simulink model "rzs10thnew2021b"  (R2021b)
settings: Solver=FixedStepDiscrete  StartTime=0.0  StopTime=10.0  FixedStep=0.001  RelTol=1e-3  EnableMultiTasking=on
values from neighbouring files (symbols this model uses):
  F = 0.0    [rzdatabase.sldd]
  T = 1.0    [rzdatabase.sldd]
libraries: simulink x143, hdlsllib x95, spsEdgeDetectorLib x3
(part 1 of 3)
settings Model: DataDictionary=rzdatabase.sldd  Creator=icemi  LastModifiedBy=LENOVO
settings SolverCC: PositivePriorityOrder=on
settings OptimizationCC: DefaultParameterBehavior=Inlined  EnhancedBackFolding=on  PassReuseOutputArgsAs=Individual arguments  ZeroExternalMemoryAtStartup=off  ZeroInternalMemoryAtStartup=off  MaxStackSize=64  OptimizeBlockOrder=speed  DifferentSizesBufferReuse=on  OptimizationCustomize=off  EfficientTunableParamExpr=on
settings DebuggingCC: ParameterTunabilityLossMsg=error
settings HardwareCC: ProdBitPerPointer=32  ProdBitPerSizeT=32  ProdBitPerPtrDiffT=32  ProdLargestAtomicInteger=Long  ProdLargestAtomicFloat=Double  ProdWordSize=32  ProdHWDeviceType=NXP->Cortex-M4  HardwareBoardFeatureSet=SoCBlockset
settings ModelReferenceCC: ModelReferenceNumInstancesAllowed=Single
settings SFSimCC: MATLABDynamicMemAlloc=off
settings RTWCC: Description=Embedded Coder  SystemTargetFile=ert.tlc  PackageGeneratedCodeAndArtifacts=on  TemplateMakefile=ert_default_tmf
settings CodeAppCC: ForceParamTrailComments=on  IgnoreCustomStorageClasses=off  OperatorAnnotations=on  SimulinkDataObjDesc=on  SFDataObjDesc=on  InsertBlockDesc=on
settings ERTTargetCC: InlinedParameterPlacement=NonHierarchical  ERTCustomFileTemplate=example_file_process.tlc

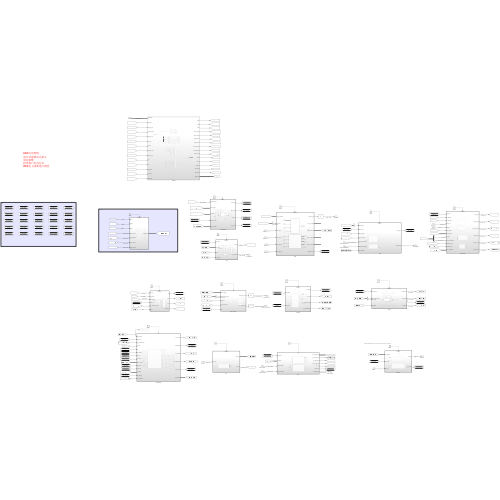
[thumbnail: Simulink's stored preview of the top-level diagram]
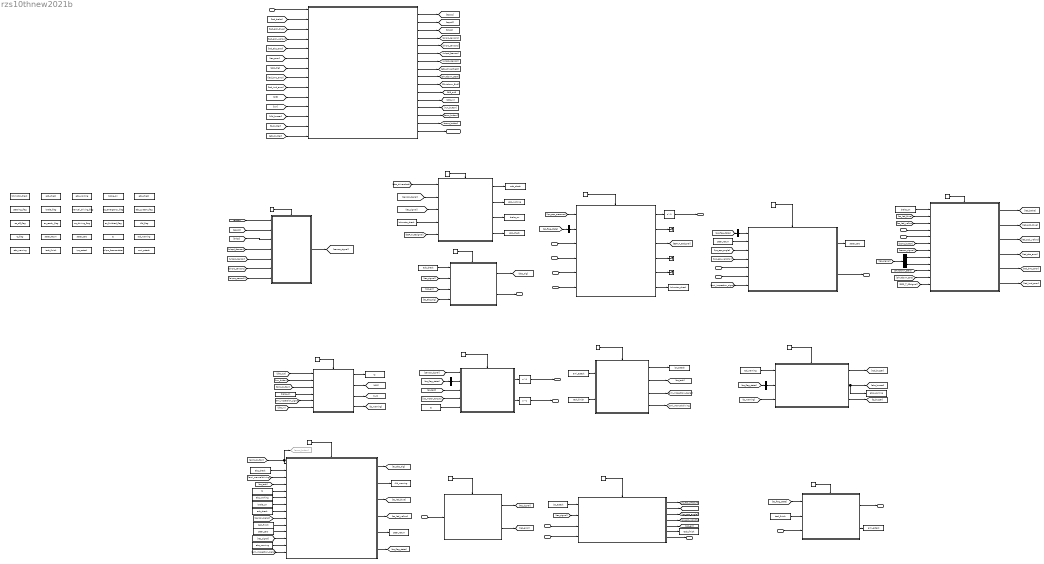
== system rzs10thnew2021b ==
  note: VCU发送状态机运行状态以及无人任务结束，接收无人任务选择
  note: EBS灯的逻辑
      | 油压传感器改为报文
      | 制动报警
      | 检查接口有没有多
      | RES定义重新建立模型
  note: 车身域
  note: 内存
  bms_error : Inport
  imd_error : Inport  Port=2
  ESP_T_01 : Inport  Port=3
  ESP_T_03 : Inport  Port=4
  ESP_T_06 : Inport  Port=5
  ESP_T_07 : Inport  Port=6
  canb_epssendmsg1 : Inport  Port=7
  canb_epssendmsg2 : Inport  Port=8
  res_msg : Inport  Port=9
  canb_ipctsmsg1 : Inport  Port=10
  canb_ipctsmsg2 : Inport  Port=11
  AMI_Tx : Inport  Port=12
  Input : Inport  Port=13  OutDataTypeStr=Bus: VCU_IN_PAR
  10ms{,1..13} (14 alike) : simulink/Ports & Subsystems/Function-Call Generator  sample_time=0.01  numberOfIterations=1  DisallowWideOutput=off
  AMI_CAN : Subsystem  TreatAsAtomicUnit=on
  ASB_Selfcheck : Subsystem  TreatAsAtomicUnit=on
  AS_AMI : Subsystem  TreatAsAtomicUnit=on
  AS_Stateflow : Subsystem  TreatAsAtomicUnit=on
  Bus Selector : BusSelector  OutputSignals=manual_driving_flag
  Bus Selector1 : BusSelector  OutputSignals=as_emergency_flag
  Bus Selector2 : BusSelector  OutputSignals=brake_flag
  Bus Selector3 : BusSelector  OutputSignals=steering_flag
  Bus Selector6 : BusSelector  OutputSignals=res_stop,res_communication
  Buzzer : Subsystem  TreatAsAtomicUnit=on
  Data Store Memory : DataStoreMemory  DataStoreName=brkmotor_check  WriteAfterWriteMsg=warning  ShowAdditionalParam=off
  Data Store Memory1 : DataStoreMemory  DataStoreName=asb_check  WriteAfterWriteMsg=warning  ShowAdditionalParam=off
  Data Store Memory10 : DataStoreMemory  DataStoreName=as_ready_flag  WriteAfterWriteMsg=warning  ShowAdditionalParam=off
  Data Store Memory11 : DataStoreMemory  DataStoreName=ts  WriteAfterWriteMsg=warning  ShowAdditionalParam=off
  Data Store Memory12 : DataStoreMemory  DataStoreName=r2d_warning  WriteAfterWriteMsg=warning  ShowAdditionalParam=off
  Data Store Memory13 : DataStoreMemory  DataStoreName=ts_flag  WriteAfterWriteMsg=warning  ShowAdditionalParam=off
  Data Store Memory14 : DataStoreMemory  DataStoreName=steer_return  WriteAfterWriteMsg=warning  ShowAdditionalParam=off
  Data Store Memory15 : DataStoreMemory  DataStoreName=as_off_flag  WriteAfterWriteMsg=warning  ShowAdditionalParam=off
  Data Store Memory16 : DataStoreMemory  DataStoreName=as_emergency_flag  WriteAfterWriteMsg=warning  ShowAdditionalParam=off
  Data Store Memory17 : DataStoreMemory  DataStoreName=as_driving_flag  WriteAfterWriteMsg=warning  ShowAdditionalParam=off
  Data Store Memory18 : DataStoreMemory  DataStoreName=r2d_flag  WriteAfterWriteMsg=warning  ShowAdditionalParam=off
  Data Store Memory19 : DataStoreMemory  DataStoreName=as_finished_flag  WriteAfterWriteMsg=warning  ShowAdditionalParam=off
  Data Store Memory2 : DataStoreMemory  DataStoreName=ebs_working  WriteAfterWriteMsg=warning  ShowAdditionalParam=off
  Data Store Memory20 : DataStoreMemory  DataStoreName=ebs_warning  WriteAfterWriteMsg=warning  ShowAdditionalParam=off
  Data Store Memory21 : DataStoreMemory  DataStoreName=task_finish  WriteAfterWriteMsg=warning  ShowAdditionalParam=off
  Data Store Memory22 : DataStoreMemory  DataStoreName=ipc_astask  WriteAfterWriteMsg=warning  ShowAdditionalParam=off
  Data Store Memory23 : DataStoreMemory  DataStoreName=ami_astask  WriteAfterWriteMsg=warning  ShowAdditionalParam=off
  Data Store Memory24 : DataStoreMemory  DataStoreName=oilprs_frsensordata  WriteAfterWriteMsg=warning  ShowAdditionalParam=off
  Data Store Memory3 : DataStoreMemory  DataStoreName=brake_on  WriteAfterWriteMsg=warning  ShowAdditionalParam=off
  Data Store Memory4 : DataStoreMemory  DataStoreName=ebs_check  WriteAfterWriteMsg=warning  ShowAdditionalParam=off
  Data Store Memory5 : DataStoreMemory  DataStoreName=steering_flag  WriteAfterWriteMsg=warning  ShowAdditionalParam=off
  Data Store Memory6 : DataStoreMemory  DataStoreName=brake_flag  WriteAfterWriteMsg=warning  ShowAdditionalParam=off
  Data Store Memory7 : DataStoreMemory  DataStoreName=manual_driving_flag  WriteAfterWriteMsg=warning  ShowAdditionalParam=off
  Data Store Memory8 : DataStoreMemory  DataStoreName=ebs_system_flag  WriteAfterWriteMsg=warning  ShowAdditionalParam=off
  Data Store Memory9 : DataStoreMemory  DataStoreName=steer_zero  WriteAfterWriteMsg=warning  ShowAdditionalParam=off
  Data Store Read : DataStoreRead  DataStoreName=brkmotor_check  IndexOptions=Index vector (dialog)  Indices=1  OutputSizes=1
  Data Store Read1 : DataStoreRead  DataStoreName=asb_check  IndexOptions=Index vector (dialog)  Indices=1  OutputSizes=1
  Data Store Read10 : DataStoreRead  DataStoreName=steer_zero  IndexOptions=Index vector (dialog)  Indices=1  OutputSizes=1
  Data Store Read11 : DataStoreRead  DataStoreName=ebs_warning  IndexOptions=Index vector (dialog)  Indices=1  OutputSizes=1
  Data Store Read12 : DataStoreRead  DataStoreName=task_finish  IndexOptions=Index vector (dialog)  Indices=1  OutputSizes=1
  Data Store Read13 : DataStoreRead  DataStoreName=brake_on  IndexOptions=Index vector (dialog)  Indices=1  OutputSizes=1
  Data Store Read14 : DataStoreRead  DataStoreName=ami_astask  IndexOptions=Index vector (dialog)  Indices=1  OutputSizes=1
  Data Store Read15 : DataStoreRead  DataStoreName=ts  IndexOptions=Index vector (dialog)  Indices=1  OutputSizes=1
  Data Store Read16 : DataStoreRead  DataStoreName=task_finish  IndexOptions=Index vector (dialog)  Indices=1  OutputSizes=1
  Data Store Read17 : DataStoreRead  DataStoreName=ipc_astask  IndexOptions=Index vector (dialog)  Indices=1  OutputSizes=1
  Data Store Read18 : DataStoreRead  DataStoreName=task_finish  IndexOptions=Index vector (dialog)  Indices=1  OutputSizes=1
  Data Store Read2 : DataStoreRead  DataStoreName=steer_return  IndexOptions=Index vector (dialog)  Indices=1  OutputSizes=1
  Data Store Read3 : DataStoreRead  DataStoreName=r2d_warning  IndexOptions=Index vector (dialog)  Indices=1  OutputSizes=1
  Data Store Read4 : DataStoreRead  DataStoreName=ebs_check  IndexOptions=Index vector (dialog)  Indices=1  OutputSizes=1
  Data Store Read5 : DataStoreRead  DataStoreName=brake_on  IndexOptions=Index vector (dialog)  Indices=1  OutputSizes=1
  Data Store Read6 : DataStoreRead  DataStoreName=ts  IndexOptions=Index vector (dialog)  Indices=1  OutputSizes=1
  Data Store Read7 : DataStoreRead  DataStoreName=ebs_working  IndexOptions=Index vector (dialog)  Indices=1  OutputSizes=1
  Data Store Read8 : DataStoreRead  DataStoreName=brake_on  IndexOptions=Index vector (dialog)  Indices=1  OutputSizes=1
  Data Store Read9 : DataStoreRead  DataStoreName=asb_check  IndexOptions=Index vector (dialog)  Indices=1  OutputSizes=1
  Data Store Write : DataStoreWrite  DataStoreName=asb_check  IndexOptions=Index vector (dialog)  Indices=1  OutputSizes=1
  Data Store Write1 : DataStoreWrite  DataStoreName=ebs_working  IndexOptions=Index vector (dialog)  Indices=1  OutputSizes=1
  Data Store Write10 : DataStoreWrite  DataStoreName=ipc_astask  IndexOptions=Index vector (dialog)  Indices=1  OutputSizes=1
  Data Store Write11 : DataStoreWrite  DataStoreName=task_finish  IndexOptions=Index vector (dialog)  Indices=1  OutputSizes=1
  Data Store Write12 : DataStoreWrite  DataStoreName=ami_astask  IndexOptions=Index vector (dialog)  Indices=1  OutputSizes=1
  Data Store Write2 : DataStoreWrite  DataStoreName=brake_on  IndexOptions=Index vector (dialog)  Indices=1  OutputSizes=1
  Data Store Write3 : DataStoreWrite  DataStoreName=ebs_check  IndexOptions=Index vector (dialog)  Indices=1  OutputSizes=1
  Data Store Write4 : DataStoreWrite  DataStoreName=brkmotor_check  IndexOptions=Index vector (dialog)  Indices=1  OutputSizes=1
  Data Store Write5 : DataStoreWrite  DataStoreName=steer_zero  IndexOptions=Index vector (dialog)  Indices=1  OutputSizes=1
  Data Store Write6 : DataStoreWrite  DataStoreName=ts  IndexOptions=Index vector (dialog)  Indices=1  OutputSizes=1
  Data Store Write7 : DataStoreWrite  DataStoreName=ebs_warning  IndexOptions=Index vector (dialog)  Indices=1  OutputSizes=1
  Data Store Write8 : DataStoreWrite  DataStoreName=r2d_warning  IndexOptions=Index vector (dialog)  Indices=1  OutputSizes=1
  Data Store Write9 : DataStoreWrite  DataStoreName=steer_return  IndexOptions=Index vector (dialog)  Indices=1  OutputSizes=1
  Delay : Delay  DelayLength=1  InputProcessing=Columns as channels (frame based)
  Delay1 : Delay  DelayLength=1  InputProcessing=Columns as channels (frame based)
  Delay2 : Delay  DelayLength=1  InputProcessing=Columns as channels (frame based)
  EBS : Subsystem  TreatAsAtomicUnit=on
  EPS : Subsystem
  ESP : Subsystem
  Goto27 : Goto  Commented=on  GotoTag=asms_button
  IPC : Subsystem  TreatAsAtomicUnit=on
  LED_Control : Subsystem
  Motor_Control : Subsystem  TreatAsAtomicUnit=on
  Res : Subsystem
  Sensor_Signal : Subsystem  TreatAsAtomicUnit=on
  TS_Activation : Subsystem  TreatAsAtomicUnit=on
  Terminator : Terminator
  Terminator2 : Terminator
  Terminator3 : Terminator
  analysis : Subsystem
  ESP_R_00 : Outport
  ebs_watchdog : Outport  Port=2
  canb_epsmsg : Outport  Port=3
  canb_ipcrxmsg : Outport  Port=4
  cana_motor_cmd : Outport  Port=5
  cana_motor_cmd3 : Outport  Port=6
  AMI_RX : Outport  Port=7
  Output : Outport  Port=8
  wires:
  10ms/1 -> Sensor_Signal/Trigger
  [apps1] -> Sensor_Signal/1(apps1)  "apps1"
  [apps2] -> Sensor_Signal/2(apps2)  "apps2"
  [brkps] -> Sensor_Signal/3(brkps)  "brkps"
  [wlspd_fsensor] -> Sensor_Signal/4(wlspd_fsensor)  "wlspd_fsensor"
  [wlspd_rsensor] -> Sensor_Signal/5(wlspd_hsensor)  "wlspd_hsensor"
  [airprs_sensor1] -> Sensor_Signal/6(airprs_sensor1)  "airprs_sensor1"
  10ms1/1 -> TS_Activation/Trigger
  [di8_out] -> TS_Activation/1(di8_out)  "di8_out"
  [asms_button] -> Goto27/1, AS_Stateflow/1(asms_button)  "asms_button"
  Data Store Read4/1 -> AS_Stateflow/2(ebs_check)
  [as_task] -> AS_Stateflow/4(as_task)
  Data Store Read6/1 -> AS_Stateflow/5(ts)
  Data Store Read11/1 -> AS_Stateflow/13(ebs_warning)
  Data Store Read7/1 -> AS_Stateflow/6(ebs_working)
  Data Store Read8/1 -> AS_Stateflow/7(brake_on)
  Data Store Read9/1 -> AS_Stateflow/8(asb_check)
  Data Store Read10/1 -> AS_Stateflow/11(steer_zero)
  Data Store Read18/1 -> AS_Stateflow/10(task_finish)
  AS_Stateflow/1(as_ebs_trig) -> [as_ebs_trig]
  AS_Stateflow/2(r2d_warning) -> Data Store Write8/1
  AS_Stateflow/3(as_led_blue) -> [as_led_blue]
  AS_Stateflow/4(as_led_yellow) -> [as_led_yellow]
  AS_Stateflow/5(steer_return) -> Data Store Write9/1
  10ms3/1 -> ASB_Selfcheck/Trigger
  [ebs_drivercheck] -> ASB_Selfcheck/1(ebs_drivercheck)  "ebs_drivercheck"
  [sensor_signal] -> ASB_Selfcheck/2(sensor_signal)
  [airprs_sensor2] -> Sensor_Signal/7(airprs_sensor2)  "airprs_sensor2"
  10ms4/1 -> Motor_Control/Trigger
  Bus Selector/1 -> Motor_Control/2(manual_driving_flag)  "<manual_driving_flag>"
  [as_task] -> Motor_Control/3(as_task)
  [ipc_motor_torque] -> Motor_Control/4(ipc_motor_torque)
  10ms5/1 -> AS_AMI/Trigger
  Data Store Read16/1 -> AS_AMI/2(task_finish)
  10ms6/1 -> AS_Stateflow/Trigger
  AS_AMI/1(ipc_astask) -> Data Store Write10/1
  AS_AMI/2(as_task) -> [as_task]
  [tsms_button] -> TS_Activation/3(tsms_button)  "tsms_button"
  TS_Activation/1(ts) -> Data Store Write6/1
  EBS/1(ebs_trig) -> [ebs_trig]  "ebs_trig"
  Data Store Read1/1 -> EBS/1(asb_check)
  EBS/2(ebs_watchdog) -> ebs_watchdog/1  "ebs_watchdog"
  [ipc_err] -> EBS/3(ipc_err)
  10ms7/1 -> EBS/Trigger
  10ms8/1 -> ESP/Trigger
  10ms9/1 -> EPS/Trigger
  Res/1(res_signal) -> [res_signal]
  10ms10/1 -> Res/Trigger
  [res_signal] -> AS_Stateflow/12(res_signal)
  [res_signal] -> EBS/2(res_signal)
  [ipc_esp_pressure] -> ESP/1(ipc_esp_pressure)
  ESP/6(brkmotor_check) -> Data Store Write4/1
  10ms11/1 -> IPC/Trigger
  Data Store Read17/1 -> IPC/1(ipc_astask)
  [res_signal] -> IPC/2(res_signal)
  IPC/1(ipc_esp_pressure) -> [ipc_esp_pressure]
  IPC/3(ipc_eps_angle) -> [ipc_eps_angle]
  IPC/4(ipc_eps_velocity) -> [ipc_eps_velocity]
  IPC/5(ipc_err) -> [ipc_err]
  IPC/6(task_finish) -> Data Store Write11/1
  IPC/2(ipc_motor_torque) -> [ipc_motor_torque]
  LED_Control/1(led_brake) -> [led_brake]  "led_brake"
  10ms2/1 -> LED_Control/Trigger
  [as_led_yellow] -> LED_Control/3(as_led_yellow)
  LED_Control/4(led_ebs_error) -> [led_ebs_error]  "led_ebs_error"
  LED_Control/6(led_imd_error) -> [led_imd_error]  "led_imd_error"
  LED_Control/5(led_bms_error) -> [led_bms_error]  "led_bms_error"
  [as_led_blue] -> LED_Control/2(as_led_blue)
  LED_Control/2(led_assi_blue) -> [led_assi_blue]  "led_assi_blue"
  LED_Control/3(led_assi_yellow) -> [led_assi_yellow]  "led_assi_yellow"
  bms_error/1 -> LED_Control/4(bms_error)  "bms_error"
  imd_error/1 -> LED_Control/5(imd_error)  "imd_error"
  [as_ebs_trig] -> EBS/4(as_ebs_trig)
  10ms12/1 -> Buzzer/Trigger
  Data Store Read3/1 -> Buzzer/1(r2d_warning)
  Buzzer/1(r2d_buzzer) -> [r2d_buzzer]  "r2d_buzzer"
  Buzzer/2(ebs_buzzer) -> [ebs_buzzer], Data Store Write7/1  "ebs_buzzer"
  Data Store Read5/1 -> TS_Activation/4(brake_on)
  [asms_button] -> LED_Control/6(asms_button)
  AS_Stateflow/6(as_flag_state) -> [as_flag_state]
  [as_flag_state] -> Bus Selector/1
  [as_flag_state] -> Bus Selector1/1
  Bus Selector1/1 -> Buzzer/2(as_emergency_flag)  "<as_emergency_flag>"
  [as_flag_state] -> Bus Selector2/1
  Bus Selector2/1 -> ESP/2(brake_flag)  "<brake_flag>"
  [as_flag_state] -> Bus Selector3/1
  ESP_T_01/1 -> ESP/3(canb_esp_t01)  "ESP_T_01"
  ESP_T_03/1 -> ESP/4(canb_esp_t03)  "ESP_T_03"
  ESP_T_06/1 -> ESP/5(canb_esp_t06)  "ESP_T_06"
  ESP_T_07/1 -> ESP/6(canb_esp_t07)  "ESP_T_07"
  ESP/2(ESP_T_01sigal) -> Terminator/1
  ESP/3(ESP_T_03signal) -> [ESP_T_03signal]
  ESP/4(ESP_T_06signal) -> Terminator2/1
  ESP/5(ESP_T_07signal) -> Terminator3/1
  [ipc_eps_angle] -> EPS/3(ipc_eps_angle)
  [ipc_eps_velocity] -> EPS/4(ipc_eps_velocity)
  Data Store Read2/1 -> EPS/2(steer_return)
  Bus Selector3/1 -> EPS/1(steering_flag)  "<steering_flag>"
  EPS/1(steer_zero) -> Data Store Write5/1
  EPS/2(canb_epsmsg) -> canb_epsmsg/1  "canb_epsmsg"
  canb_epssendmsg1/1 -> EPS/5(canb_epssendmsg1)  "canb_epssendmsg1"
  canb_epssendmsg2/1 -> EPS/6(canb_epssendmsg2)  "canb_epssendmsg2"
  res_msg/1 -> Res/1(res_msg)  "res_msg"
  canb_ipctsmsg2/1 -> IPC/4(canb_ipctsmsg2)  "canb_ipctsmsg2"
  canb_ipctsmsg1/1 -> IPC/3(canb_ipctsmsg1)  "canb_ipctsmsg1"
  IPC/7(canb_ipcrxmsg) -> canb_ipcrxmsg/1  "canb_ipcrxmsg"
  [run_button] -> TS_Activation/2(run_button)  "run_button"
  Data Store Read/1 -> ASB_Selfcheck/4(brkmotor_check)
  ASB_Selfcheck/1(asb_check) -> Data Store Write/1
  ASB_Selfcheck/2(ebs_working) -> Data Store Write1/1
  ASB_Selfcheck/3(brake_on) -> Data Store Write2/1
  ASB_Selfcheck/4(ebs_check) -> Data Store Write3/1
  Data Store Read13/1 -> LED_Control/1(brake_on)
  Data Store Read15/1 -> Motor_Control/5(ts)
  [ami_inspection_signal] -> TS_Activation/5(ami_inspection_signal)
  [di8_in] -> TS_Activation/6(di8_in)  "di8_in"
  [ami_inspection_signal] -> EPS/7(ami_inspection)
  [res_signal] -> ASB_Selfcheck/3(res_signal)
  [res_signal] -> Bus Selector6/1
  Bus Selector6/1 -> LED_Control/8(res_stop)  "<res_stop>"
  Bus Selector6/2 -> LED_Control/9(res_communication)  "<res_communication>"
  [Shutdown_Start] -> LED_Control/10(Shutdown_Start)
  [Shutdown_End] -> LED_Control/11(Shutdown_End)
  [sensor_signal] -> LED_Control/7(sensor_signal)
  [ami_inspection_signal] -> AS_Stateflow/14(ami_inspection)
  [sensor_signal] -> Motor_Control/1(sensor_signal)
  [sensor_signal] -> AS_Stateflow/9(sensor_signal)
  Sensor_Signal/1(sensor_signal) -> [sensor_signal]
  [ESP_T_03signal] -> ASB_Selfcheck/5(ESP_T_03signal)
  [ESP_T_03signal] -> LED_Control/12(ESP_T_03signal)
  AS_AMI/3(ami_inspection_signal) -> [ami_inspection_signal]
  TS_Activation/2(di8) -> [di8]
  TS_Activation/3(run) -> [run]
  AMI_Tx/1 -> AMI_CAN/3(AMI_Tx)  "AMI_Tx"
  [as_flag_state] -> AMI_CAN/1(as_flag_state)
  Data Store Read12/1 -> AMI_CAN/2(task_finish)
  AMI_CAN/1(AMI_RX) -> AMI_RX/1  "AMI_Rx"
  Data Store Read14/1 -> AS_AMI/1(ami_astask)
  10ms13/1 -> AMI_CAN/Trigger
  AMI_CAN/2(ami_astask) -> Data Store Write12/1
  [ts_warning] -> Buzzer/3(ts_warning)
  TS_Activation/4(ts_warning) -> [ts_warning]
  Buzzer/3(ts_buzzer) -> [ts_buzzer]  "ts_buzzer"
  AS_AMI/4(ami_manualdriving) -> [ami_manualdriving]
  [ami_manualdriving] -> AS_Stateflow/3(ami_manualdriving)
  Res/2(res_error) -> [res_error]  "res_error"
  [led_brake] -> analysis/2(led_brake)
  [led_assi_blue] -> analysis/3(led_assi_blue)
  [led_assi_yellow] -> analysis/4(led_assi_yellow)
  [led_ebs_error] -> analysis/5(led_ebs_error)
  [res_error] -> analysis/6(res_error)
  [ebs_trig] -> analysis/7(ebs_trig)
  [led_bms_error] -> analysis/8(led_bms_error)
  [led_imd_error] -> analysis/9(led_imd_error)
  [di8] -> analysis/10(di8)
  [run] -> analysis/11(run)
  [r2d_buzzer] -> analysis/12(r2d_buzzer)
  [ts_buzzer] -> analysis/13(ts_buzzer)
  [ebs_buzzer] -> analysis/14(ebs_buzzer)
  analysis/1(Output) -> [apps1]
  analysis/2(Output1) -> [apps2]
  analysis/5(Output3) -> [airprs_sensor2]
  analysis/6(Output4) -> [wlspd_fsensor]
  analysis/7(Output5) -> [wlspd_rsensor]
  analysis/3(Output6) -> [brkps]
  analysis/4(Output2) -> [airprs_sensor1]
  analysis/8(Output7) -> [ebs_drivercheck]
  analysis/9(Output8) -> [Shutdown_Start]
  analysis/10(Output9) -> [Shutdown_End]
  analysis/11(Output10) -> [di8_out]
  analysis/12(Output11) -> [di8_in]
  analysis/13(Output12) -> [run_button]
  analysis/14(Output13) -> [tsms_button]
  analysis/15(Output14) -> [asms_button]
  analysis/16(Output15) -> Output/1  "digital_output"
  Input/1 -> analysis/1(digital_input)  "digital_input"
  ESP/1(canb_esp_r00) -> Delay/1
  Delay/1 -> ESP_R_00/1  "ESP_R_00"
  Motor_Control/2(cana_motor_cmd3) -> Delay2/1
  Delay2/1 -> cana_motor_cmd3/1  "cana_motor_cmd3"
  Motor_Control/1(cana_motor_cmd) -> Delay1/1
  Delay1/1 -> cana_motor_cmd/1  "cana_motor_cmd"

== system rzs10thnew2021b/AMI_CAN ==
  as_flag_state : Inport
  task_finish : Inport  Port=2
  AMI_Tx : Inport  Port=3
  function : TriggerPort  TriggerType=function-call  VariantControl=(inherit)
  AMI_Receivemsg : Subsystem
  AMI_Transmitmsg : Subsystem  Commented=on
  Terminator5 : Terminator  Commented=on
  AMI_RX : Outport
  ami_astask : Outport  Port=2
  wires:
  AMI_Receivemsg/1(ami_astask) -> ami_astask/1
  AMI_Tx/1 -> AMI_Receivemsg/1(AMI_Tx)
  as_flag_state/1 -> AMI_Transmitmsg/1(as_flag_state)
  task_finish/1 -> AMI_Transmitmsg/2(task_finish)
  AMI_Receivemsg/2(Output) -> AMI_RX/1

== system rzs10thnew2021b/ASB_Selfcheck ==
  note: 制动相关压力是否支持正常工作
  note: EBS驱动上电
  note: 前气路是否有压力
  note: EBS板子是否上电
  note: 工作后EBS手动阀是否释放
  ebs_drivercheck : Inport
  sensor_signal : Inport  Port=2
  res_signal : Inport  Port=3
  brkmotor_check : Inport  Port=4
  ESP_T_03signal : Inport  Port=5
  function : TriggerPort  TriggerType=function-call  VariantControl=(inherit)
  Brake_Sensor_Check : Subsystem
  Bus Selector : BusSelector  OutputSignals=airprs_sensor1,airprs_sensor2
  Bus Selector1 : BusSelector  OutputSignals=res_check
  Bus Selector2 : BusSelector  OutputSignals=oilprs_flsensor,oilprs_frsensor,oilprs_rlsensor,oilprs_rrsensor
  Compare To Constant : simulink/Logic and Bit Operations/Compare To Constant  relop===  const=0  OutDataTypeStr=boolean
  Compare To Constant1 : simulink/Logic and Bit Operations/Compare To Constant  relop=>=  const=0.74  OutDataTypeStr=boolean
  EBS_On_Check : Subsystem
  Logical Operator : Logic  Inputs=4  AllPortsSameDT=off  OutDataTypeStr=boolean
  Logical Operator1 : Logic  Inputs=3  AllPortsSameDT=off  OutDataTypeStr=boolean
  asb_check : Outport
  ebs_working : Outport  Port=2
  brake_on : Outport  Port=3
  ebs_check : Outport  Port=4
  wires:
  sensor_signal/1 -> Bus Selector/1
  Bus Selector/1 -> Compare To Constant1/1, Brake_Sensor_Check/1(airprs_sensor1)  "<airprs_sensor1>"
  Brake_Sensor_Check/1(brksensor_check) -> Logical Operator/2
  ebs_drivercheck/1 -> Logical Operator/1, Logical Operator1/2
  brkmotor_check/1 -> Logical Operator/4
  Logical Operator/1 -> asb_check/1
  Bus Selector/2 -> EBS_On_Check/1(airprs_sensor2)  "<airprs_sensor2>"
  EBS_On_Check/1(ebs_working) -> ebs_working/1, [ebs_working]
  Brake_Sensor_Check/2(brake_on) -> brake_on/1
  Compare To Constant/1 -> Logical Operator1/1
  [ebs_working] -> Compare To Constant/1
  Compare To Constant1/1 -> Logical Operator1/3
  Logical Operator1/1 -> ebs_check/1
  res_signal/1 -> Bus Selector1/1
  Bus Selector1/1 -> Logical Operator/3  "<res_check>"
  ESP_T_03signal/1 -> Bus Selector2/1
  Bus Selector2/1 -> Brake_Sensor_Check/2(oilprs_frsensor)  "<oilprs_flsensor>"
  Bus Selector2/2 -> Brake_Sensor_Check/3(oilprs_rrsensor)  "<oilprs_frsensor>"
  Bus Selector2/3 -> Brake_Sensor_Check/4(oilprs_flsensor)  "<oilprs_rlsensor>"
  Bus Selector2/4 -> Brake_Sensor_Check/5(oilprs_rlsensor)  "<oilprs_rrsensor>"

== system rzs10thnew2021b/AS_AMI ==
  ami_astask : Inport
  task_finish : Inport  Port=2
  function : TriggerPort  TriggerType=function-call  VariantControl=(inherit)
  Chart : Stateflow chart  TreatAsAtomicUnit=on
  Constant : Constant  Value=0  OutDataTypeStr=boolean
  Constant1 : Constant  OutDataTypeStr=boolean
  Constant2 : Constant  OutDataTypeStr=boolean
  Constant3 : Constant  Value=0  OutDataTypeStr=boolean
  Switch : Switch  Criteria=u2 > Threshold
  Switch1 : Switch  Threshold=5
  ipc_astask : Outport
  as_task : Outport  Port=2
  ami_inspection_signal : Outport  Port=3
  ami_manualdriving : Outport  Port=4
  wires:
  Chart/1(ipc_astask) -> Switch1/2, ipc_astask/1, Switch/2
  task_finish/1 -> Chart/2(task_finish)
  ami_astask/1 -> Chart/1(ami_astask)
  Chart/2(ami_inspection_signal) -> ami_inspection_signal/1
  Switch/1 -> as_task/1
  Constant/1 -> Switch/3
  Constant1/1 -> Switch/1
  Constant2/1 -> Switch1/1
  Constant3/1 -> Switch1/3
  Switch1/1 -> ami_manualdriving/1

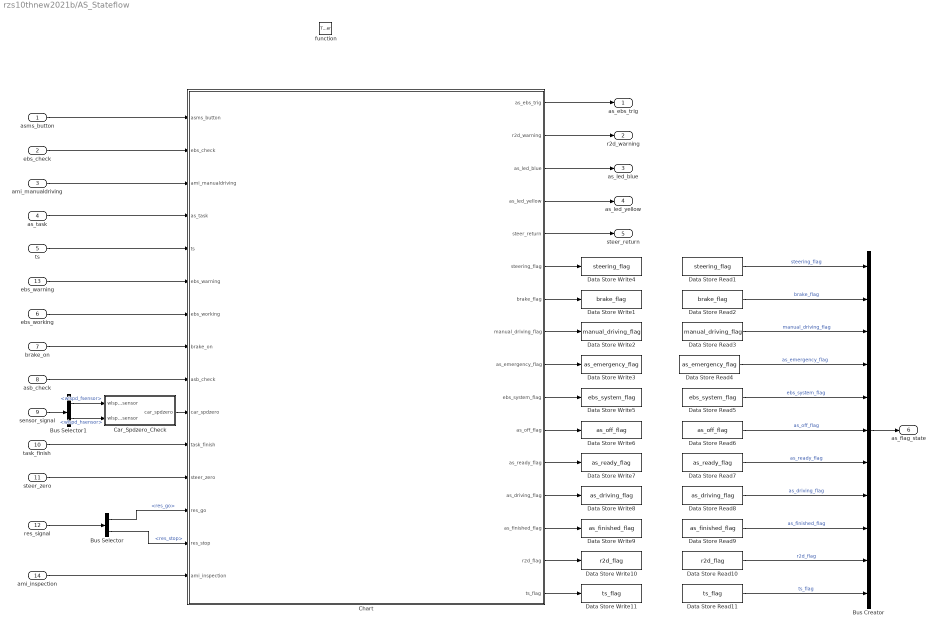
== system rzs10thnew2021b/AS_Stateflow ==
  asms_button : Inport
  ebs_check : Inport  Port=2
  ami_manualdriving : Inport  Port=3
  as_task : Inport  Port=4
  ts : Inport  Port=5
  ebs_working : Inport  Port=6
  brake_on : Inport  Port=7
  asb_check : Inport  Port=8
  sensor_signal : Inport  Port=9
  task_finish : Inport  Port=10
  steer_zero : Inport  Port=11
  res_signal : Inport  Port=12
  ebs_warning : Inport  Port=13
  ami_inspection : Inport  Port=14
  function : TriggerPort  TriggerType=function-call  VariantControl=(inherit)
  Bus Creator : BusCreator  Inputs=11
  Bus Selector : BusSelector  OutputSignals=res_go,res_stop
  Bus Selector1 : BusSelector  OutputSignals=wlspd_fsensor,wlspd_hsensor
  Car_Spdzero_Check : Subsystem
  Chart : Stateflow chart  TreatAsAtomicUnit=on
      settings: PortSchema="{\"entries\":[{\"content\":{\"sides\":[{\"content\":{\"connectorIds\":[\"In1\",\"In2\",\"In3\",\"In4\",\"In5\",\"In6\",\"In7\",\"In8\",\"In9\",\"In10\",\"In11\",\"In13\",\"In12\",\"In14\",\"In15\"]},\"type\":\"ConnectorPlacement.EquallySpacedRectSide\",\"uuid\":\"5ff7b962-0009-43e2-919e-affd8aae6d9f\"},{\"content\":{\"connectorIds\":[\"Out1\",\"Out2\",\"Out3\",\"Out4\",\"Out5\",\"Out6\",\"Out7\",\"Out8\",\"Out9\",\"Out10\",\"Out11\",\"Out12\",\"Out13\",\"Out14\",\"Out15\",\"Out16\"],\"side\":\"RIGHT\"},\"type\":\"ConnectorPlacement.EquallySpacedRectSide\",\"uuid\":\"8fbd6d23-6f6b-4ff9-8347-09da63d88237\"},{\"content\":{\"side\":\"TOP\"},\"type\":\"ConnectorPlacement.EquallySpacedRectSide\",\"uuid\":\"5115a408-a5f8-47e8-8fa4-cf60e643eb64\"}]},\"type\":\"ConnectorPlacement.EquallySpacedConnector\",\"uuid\":\"6f9469b9-2522-48d3-80b2-5e824d353f63\"}],\"packageUris\":[\"http://schema.mathworks.com/mf0/Connector/R2020b\"],\"version\":\"1.0\"}"
  Data Store Read1 : DataStoreRead  DataStoreName=steering_flag  IndexOptions=Index vector (dialog)  Indices=1  OutputSizes=1
  Data Store Read10 : DataStoreRead  DataStoreName=r2d_flag  IndexOptions=Index vector (dialog)  Indices=1  OutputSizes=1
  Data Store Read11 : DataStoreRead  DataStoreName=ts_flag  IndexOptions=Index vector (dialog)  Indices=1  OutputSizes=1
  Data Store Read2 : DataStoreRead  DataStoreName=brake_flag  IndexOptions=Index vector (dialog)  Indices=1  OutputSizes=1
  Data Store Read3 : DataStoreRead  DataStoreName=manual_driving_flag  IndexOptions=Index vector (dialog)  Indices=1  OutputSizes=1
  Data Store Read4 : DataStoreRead  DataStoreName=as_emergency_flag  IndexOptions=Index vector (dialog)  Indices=1  OutputSizes=1
  Data Store Read5 : DataStoreRead  DataStoreName=ebs_system_flag  IndexOptions=Index vector (dialog)  Indices=1  OutputSizes=1
  Data Store Read6 : DataStoreRead  DataStoreName=as_off_flag  IndexOptions=Index vector (dialog)  Indices=1  OutputSizes=1
  Data Store Read7 : DataStoreRead  DataStoreName=as_ready_flag  IndexOptions=Index vector (dialog)  Indices=1  OutputSizes=1
  Data Store Read8 : DataStoreRead  DataStoreName=as_driving_flag  IndexOptions=Index vector (dialog)  Indices=1  OutputSizes=1
  Data Store Read9 : DataStoreRead  DataStoreName=as_finished_flag  IndexOptions=Index vector (dialog)  Indices=1  OutputSizes=1
  Data Store Write1 : DataStoreWrite  DataStoreName=brake_flag  IndexOptions=Index vector (dialog)  Indices=1  OutputSizes=1
  Data Store Write10 : DataStoreWrite  DataStoreName=r2d_flag  IndexOptions=Index vector (dialog)  Indices=1  OutputSizes=1
  Data Store Write11 : DataStoreWrite  DataStoreName=ts_flag  IndexOptions=Index vector (dialog)  Indices=1  OutputSizes=1
  Data Store Write2 : DataStoreWrite  DataStoreName=manual_driving_flag  IndexOptions=Index vector (dialog)  Indices=1  OutputSizes=1
  Data Store Write3 : DataStoreWrite  DataStoreName=as_emergency_flag  IndexOptions=Index vector (dialog)  Indices=1  OutputSizes=1
  Data Store Write4 : DataStoreWrite  DataStoreName=steering_flag  IndexOptions=Index vector (dialog)  Indices=1  OutputSizes=1
  Data Store Write5 : DataStoreWrite  DataStoreName=ebs_system_flag  IndexOptions=Index vector (dialog)  Indices=1  OutputSizes=1
  Data Store Write6 : DataStoreWrite  DataStoreName=as_off_flag  IndexOptions=Index vector (dialog)  Indices=1  OutputSizes=1
  Data Store Write7 : DataStoreWrite  DataStoreName=as_ready_flag  IndexOptions=Index vector (dialog)  Indices=1  OutputSizes=1
  Data Store Write8 : DataStoreWrite  DataStoreName=as_driving_flag  IndexOptions=Index vector (dialog)  Indices=1  OutputSizes=1
  Data Store Write9 : DataStoreWrite  DataStoreName=as_finished_flag  IndexOptions=Index vector (dialog)  Indices=1  OutputSizes=1
  as_ebs_trig : Outport
  r2d_warning : Outport  Port=2
  as_led_blue : Outport  Port=3
  as_led_yellow : Outport  Port=4
  steer_return : Outport  Port=5
  as_flag_state : Outport  Port=6
  wires:
  asms_button/1 -> Chart/1(asms_button)
  ebs_check/1 -> Chart/2(ebs_check)
  ami_manualdriving/1 -> Chart/3(ami_manualdriving)
  as_task/1 -> Chart/4(as_task)
  ebs_working/1 -> Chart/7(ebs_working)
  brake_on/1 -> Chart/8(brake_on)
  asb_check/1 -> Chart/9(asb_check)
  task_finish/1 -> Chart/11(task_finish)
  steer_zero/1 -> Chart/13(steer_zero)
  ts/1 -> Chart/5(ts)
  Chart/1(as_ebs_trig) -> as_ebs_trig/1
  Chart/2(r2d_warning) -> r2d_warning/1
  Chart/3(as_led_blue) -> as_led_blue/1
  Chart/4(as_led_yellow) -> as_led_yellow/1
  Chart/5(steer_return) -> steer_return/1
  ebs_warning/1 -> Chart/6(ebs_warning)
  res_signal/1 -> Bus Selector/1
  Bus Selector/2 -> Chart/14(res_stop)  "<res_stop>"
  Bus Selector/1 -> Chart/12(res_go)  "<res_go>"
  sensor_signal/1 -> Bus Selector1/1
  Bus Selector1/1 -> Car_Spdzero_Check/1(wlspd_fsensor)  "<wlspd_fsensor>"
  Bus Selector1/2 -> Car_Spdzero_Check/2(wlspd_hsensor)  "<wlspd_hsensor>"
  Car_Spdzero_Check/1(car_spdzero) -> Chart/10(car_spdzero)
  Bus Creator/1 -> as_flag_state/1
  Chart/6(steering_flag) -> Data Store Write4/1
  Data Store Read1/1 -> Bus Creator/1  "steering_flag"
  Chart/7(brake_flag) -> Data Store Write1/1
  Data Store Read2/1 -> Bus Creator/2  "brake_flag"
  Chart/8(manual_driving_flag) -> Data Store Write2/1
  Data Store Read3/1 -> Bus Creator/3  "manual_driving_flag"
  Data Store Read4/1 -> Bus Creator/4  "as_emergency_flag"
  Chart/9(as_emergency_flag) -> Data Store Write3/1
  Chart/10(ebs_system_flag) -> Data Store Write5/1
  Data Store Read5/1 -> Bus Creator/5  "ebs_system_flag"
  Chart/11(as_off_flag) -> Data Store Write6/1
  Data Store Read6/1 -> Bus Creator/6  "as_off_flag"
  Chart/12(as_ready_flag) -> Data Store Write7/1
  Data Store Read7/1 -> Bus Creator/7  "as_ready_flag"
  Chart/13(as_driving_flag) -> Data Store Write8/1
  Data Store Read8/1 -> Bus Creator/8  "as_driving_flag"
  Chart/14(as_finished_flag) -> Data Store Write9/1
  Data Store Read9/1 -> Bus Creator/9  "as_finished_flag"
  Chart/15(r2d_flag) -> Data Store Write10/1
  Data Store Read10/1 -> Bus Creator/10  "r2d_flag"
  Data Store Read11/1 -> Bus Creator/11  "ts_flag"
  Chart/16(ts_flag) -> Data Store Write11/1
  ami_inspection/1 -> Chart/15(ami_inspection)

== system rzs10thnew2021b/Buzzer ==
  r2d_warning : Inport
  as_emergency_flag : Inport  Port=2
  ts_warning : Inport  Port=3
  function : TriggerPort  TriggerType=function-call  VariantControl=(inherit)
  Chart : Stateflow chart  TreatAsAtomicUnit=on
  Constant : Constant  Value=0  OutDataTypeStr=boolean
  Data Type Conversion6 : DataTypeConversion  OutDataTypeStr=boolean
  Pulse Generator : DiscretePulseGenerator  Period=100  PulseWidth=50  SampleTime=-1
  Switch : Switch  Criteria=u2 > Threshold
  r2d_buzzer : Outport
  ebs_buzzer : Outport  Port=2
  ts_buzzer : Outport  Port=3
  wires:
  r2d_warning/1 -> r2d_buzzer/1
  as_emergency_flag/1 -> Chart/1(as_emergency_flag)
  Chart/1(ebs_buzzer) -> Switch/2
  Switch/1 -> ebs_buzzer/1
  Constant/1 -> Switch/3
  Pulse Generator/1 -> Data Type Conversion6/1
  Data Type Conversion6/1 -> Switch/1
  ts_warning/1 -> ts_buzzer/1

== system rzs10thnew2021b/EBS ==
  asb_check : Inport
  res_signal : Inport  Port=2
  ipc_err : Inport  Port=3
  as_ebs_trig : Inport  Port=4
  function : TriggerPort  TriggerType=function-call  VariantControl=(inherit)
  Bus Selector : BusSelector  OutputSignals=res_check
  Data Type Conversion5 : DataTypeConversion  OutDataTypeStr=boolean
  Edge Detector : spsEdgeDetectorLib/Edge Detector  model=Falling  ic=0  Ts=-1
      settings: SourceProductBaseCode=PS
  Edge Detector1 : spsEdgeDetectorLib/Edge Detector  model=Falling  ic=0  Ts=-1
      settings: SourceProductBaseCode=PS
  Edge Detector2 : spsEdgeDetectorLib/Edge Detector  model=Falling  ic=0  Ts=-1
      settings: SourceProductBaseCode=PS
  Logical Operator : Logic  Operator=OR  Inputs=4  AllPortsSameDT=off  OutDataTypeStr=boolean
  Pulse Generator : DiscretePulseGenerator  Period=10  PulseWidth=5  SampleTime=-1
  ebs_trig : Outport
  ebs_watchdog : Outport  Port=2
  wires:
  asb_check/1 -> Edge Detector/1
  Pulse Generator/1 -> Data Type Conversion5/1
  res_signal/1 -> Bus Selector/1
  Bus Selector/1 -> Edge Detector1/1  "<res_check>"
  ipc_err/1 -> Edge Detector2/1
  Edge Detector/1 -> Logical Operator/1
  Edge Detector1/1 -> Logical Operator/2
  Edge Detector2/1 -> Logical Operator/3
  as_ebs_trig/1 -> Logical Operator/4
  Logical Operator/1 -> ebs_trig/1
  Data Type Conversion5/1 -> ebs_watchdog/1

== system rzs10thnew2021b/EPS ==
  steering_flag : Inport
  steer_return : Inport  Port=2
  ipc_eps_angle : Inport  Port=3
  ipc_eps_velocity : Inport  Port=4
  canb_epssendmsg1 : Inport  Port=5
  canb_epssendmsg2 : Inport  Port=6
  ami_inspection : Inport  Port=7
  function : TriggerPort  TriggerType=function-call  VariantControl=(inherit)
  Bus Selector : BusSelector  OutputSignals=eps_realangle
  EPS_ReceiveMsg : Subsystem
  EPS_TransmitMsg : Subsystem
  Terminator : Terminator
  steer_zero : Outport
  canb_epsmsg : Outport  Port=2
  wires:
  steering_flag/1 -> EPS_TransmitMsg/1(steering_flag)
  steer_return/1 -> EPS_TransmitMsg/2(steer_return)
  ipc_eps_angle/1 -> EPS_TransmitMsg/3(eps_wheel_angle)
  ipc_eps_velocity/1 -> EPS_TransmitMsg/4(ipc_eps_velocity)
  EPS_TransmitMsg/1(canb_epsmsg) -> canb_epsmsg/1
  EPS_TransmitMsg/2(steer_zero) -> steer_zero/1
  canb_epssendmsg1/1 -> EPS_ReceiveMsg/1(canb_epssendmsg1)
  canb_epssendmsg2/1 -> EPS_ReceiveMsg/2(canb_epssendmsg2)
  EPS_ReceiveMsg/2(canb_epssendmsg2signal) -> Terminator/1
  EPS_ReceiveMsg/1(canb_epssendmsg1signal) -> [canb_epssendmsg1signal]
  Bus Selector/1 -> EPS_TransmitMsg/5(eps_realangle)  "<eps_realangle>"
  [canb_epssendmsg1signal] -> Bus Selector/1
  ami_inspection/1 -> EPS_TransmitMsg/6(ami_inspection)

== system rzs10thnew2021b/ESP ==
  note: 可不发
  ipc_esp_pressure : Inport
  brake_flag : Inport  Port=2
  canb_esp_t01 : Inport  Port=3
  canb_esp_t03 : Inport  Port=4
  canb_esp_t06 : Inport  Port=5
  canb_esp_t07 : Inport  Port=6
  function : TriggerPort  TriggerType=function-call  VariantControl=(inherit)
  ESP_ReceiveMsg : Subsystem
  ESP_TransmitMsg : Subsystem
  checkSum : Ground
  lifeSig : Ground
  canb_esp_r00 : Outport
  ESP_T_01sigal : Outport  Port=2
  ESP_T_03signal : Outport  Port=3
  ESP_T_06signal : Outport  Port=4
  ESP_T_07signal : Outport  Port=5
  brkmotor_check : Outport  Port=6
  wires:
  ESP_ReceiveMsg/5(brkmotor_check) -> brkmotor_check/1
  brake_flag/1 -> ESP_TransmitMsg/2(brake_flag)
  ipc_esp_pressure/1 -> ESP_TransmitMsg/1(ipc_esp_pressure)
  canb_esp_t01/1 -> ESP_ReceiveMsg/1(canb_esp_t01)
  canb_esp_t07/1 -> ESP_ReceiveMsg/4(canb_esp_t07)
  canb_esp_t06/1 -> ESP_ReceiveMsg/3(canb_esp_t06)
  canb_esp_t03/1 -> ESP_ReceiveMsg/2(canb_esp_t03)
  ESP_ReceiveMsg/1(ESP_T_01sigal) -> ESP_T_01sigal/1
  ESP_ReceiveMsg/4(ESP_T_07signal) -> ESP_T_07signal/1
  ESP_ReceiveMsg/3(ESP_T_06signal) -> ESP_T_06signal/1
  ESP_ReceiveMsg/2(ESP_T_03signal) -> ESP_T_03signal/1
  checkSum/1 -> ESP_TransmitMsg/4(checkSum)
  ESP_TransmitMsg/1(canb_esp_r00) -> canb_esp_r00/1
  lifeSig/1 -> ESP_TransmitMsg/3(lifeSig)

== system rzs10thnew2021b/IPC ==
  ipc_astask : Inport
  res_signal : Inport  Port=2
  canb_ipctsmsg1 : Inport  Port=3
  canb_ipctsmsg2 : Inport  Port=4
  function : TriggerPort  TriggerType=function-call  VariantControl=(inherit)
  Bus Selector : BusSelector  OutputSignals=res_go,res_stop
  IPC_ReceiveMsg : Subsystem
  IPC_TransmitMsg : Subsystem
  ipc_esp_pressure : Outport
  ipc_motor_torque : Outport  Port=2
  ipc_eps_angle : Outport  Port=3
  ipc_eps_velocity : Outport  Port=4
  ipc_err : Outport  Port=5
  task_finish : Outport  Port=6
  canb_ipcrxmsg : Outport  Port=7
  wires:
  ipc_astask/1 -> IPC_ReceiveMsg/3(ipc_astask)
  res_signal/1 -> Bus Selector/1
  Bus Selector/1 -> IPC_ReceiveMsg/1(ipc_resgo)  "<res_go>"
  Bus Selector/2 -> IPC_ReceiveMsg/2(ipc_resstop)  "<res_stop>"
  IPC_TransmitMsg/6(task_finish) -> task_finish/1
  IPC_TransmitMsg/5(ipc_err) -> ipc_err/1
  IPC_TransmitMsg/4(ipc_eps_velocity) -> ipc_eps_velocity/1
  IPC_TransmitMsg/3(ipc_eps_angle) -> ipc_eps_angle/1
  IPC_TransmitMsg/2(ipc_motor_torque) -> ipc_motor_torque/1
  IPC_TransmitMsg/1(ipc_esp_pressure) -> ipc_esp_pressure/1
  canb_ipctsmsg2/1 -> IPC_TransmitMsg/2(canb_ipctsmsg2)
  canb_ipctsmsg1/1 -> IPC_TransmitMsg/1(canb_ipctsmsg1)
  IPC_ReceiveMsg/1(canb_ipcrxmsg) -> canb_ipcrxmsg/1

== system rzs10thnew2021b/LED_Control ==
  brake_on : Inport
  as_led_blue : Inport  Port=2
  as_led_yellow : Inport  Port=3
  bms_error : Inport  Port=4
  imd_error : Inport  Port=5
  asms_button : Inport  Port=6
  sensor_signal : Inport  Port=7
  res_stop : Inport  Port=8
  res_communication : Inport  Port=9
  Shutdown_Start : Inport  Port=10
  Shutdown_End : Inport  Port=11
  ESP_T_03signal : Inport  Port=12
  function : TriggerPort  TriggerType=function-call  VariantControl=(inherit)
  BMS_LED : Subsystem
  EBS_LED : Subsystem
  Subsystem : Subsystem
  Subsystem1 : Subsystem
  led_brake : Outport
  led_assi_blue : Outport  Port=2
  led_assi_yellow : Outport  Port=3
  led_ebs_error : Outport  Port=4
  led_bms_error : Outport  Port=5
  led_imd_error : Outport  Port=6
  wires:
  brake_on/1 -> led_brake/1
  as_led_blue/1 -> Subsystem/1(as_led_blue1)
  Subsystem/1(led_assi_blue) -> led_assi_blue/1
  Subsystem1/1(led_assi_yellow) -> led_assi_yellow/1
  as_led_yellow/1 -> Subsystem1/2(as_led_yellow)
  bms_error/1 -> BMS_LED/1(bms_error)
  imd_error/1 -> BMS_LED/2(imd_error)
  BMS_LED/1(led_bms_error) -> led_bms_error/1  "led_bms_error"
  BMS_LED/2(led_imd_error) -> led_imd_error/1  "led_imd_error"
  asms_button/1 -> Subsystem1/1(asms_button), [asms_button], Subsystem/2(asms_button)
  res_stop/1 -> EBS_LED/1(res_stop)
  res_communication/1 -> EBS_LED/2(res_communication)
  Shutdown_Start/1 -> EBS_LED/3(Shutdown_Start)
  Shutdown_End/1 -> EBS_LED/4(Shutdown_End)
  sensor_signal/1 -> EBS_LED/5(sensor_signal)
  ESP_T_03signal/1 -> EBS_LED/6(ESP_T_03signal)
  EBS_LED/1(led_ebs_error) -> led_ebs_error/1
  [asms_button] -> EBS_LED/7(asms_button)

== system rzs10thnew2021b/Motor_Control ==
  sensor_signal : Inport
  manual_driving_flag : Inport  Port=2
  as_task : Inport  Port=3
  ipc_motor_torque : Inport  Port=4
  ts : Inport  Port=5
  function : TriggerPort  TriggerType=function-call  VariantControl=(inherit)
  AS_Torque_Calculation : Subsystem  TreatAsAtomicUnit=on
  MCU1_Rx_Command : Subsystem
  MCU1_Rx_Command3 : Subsystem
  Manual_Torque_Calculation : Subsystem  TreatAsAtomicUnit=on
  Motor_Torque_Stateflow : Stateflow chart  TreatAsAtomicUnit=on
      settings: PortSchema="{\"entries\":[{\"content\":{\"sides\":[{\"content\":{\"connectorIds\":[\"In1\",\"In3\",\"In2\",\"In4\"]},\"type\":\"ConnectorPlacement.EquallySpacedRectSide\",\"uuid\":\"d9a8263c-4b6f-42da-8ac2-d6351ac22d7e\"},{\"content\":{\"connectorIds\":[\"Out1\"],\"side\":\"RIGHT\"},\"type\":\"ConnectorPlacement.EquallySpacedRectSide\",\"uuid\":\"5afddd84-d4d9-4932-bab9-0cf7e7557aa2\"},{\"content\":{\"connectorIds\":[],\"side\":\"TOP\"},\"type\":\"ConnectorPlacement.EquallySpacedRectSide\",\"uuid\":\"31244ac9-97b6-45b3-a8be-c5389c850836\"}]},\"type\":\"ConnectorPlacement.EquallySpacedConnector\",\"uuid\":\"4a9ac252-b735-4ae7-9487-f10bc9e5bec6\"}],\"packageUris\":[\"http://schema.mathworks.com/mf0/Connector/R2020b\"],\"version\":\"1.0\"}"
  cana_motor_cmd : Outport
  cana_motor_cmd3 : Outport  Port=2
  wires:
  sensor_signal/1 -> Manual_Torque_Calculation/1(sensor_signal)
  manual_driving_flag/1 -> Manual_Torque_Calculation/Enable, Motor_Torque_Stateflow/1(manual_driving_flag)
  Manual_Torque_Calculation/1(manual_torque) -> [manual_torque]
  as_task/1 -> AS_Torque_Calculation/Enable, Motor_Torque_Stateflow/2(as_task)
  ipc_motor_torque/1 -> AS_Torque_Calculation/1(ipc_motor_torque)
  AS_Torque_Calculation/1(as_torque) -> [as_torque]
  [manual_torque] -> Motor_Torque_Stateflow/3(manual_torque)
  [as_torque] -> Motor_Torque_Stateflow/4(as_torque)
  Motor_Torque_Stateflow/1(motor_torque) -> [motor_torque]
  ts/1 -> MCU1_Rx_Command/1(ts)
  [motor_torque] -> MCU1_Rx_Command/2(motor_torque)
  MCU1_Rx_Command/1(cana_motor_cmd) -> cana_motor_cmd/1
  MCU1_Rx_Command3/1(cana_motor_cmd3) -> cana_motor_cmd3/1

== system rzs10thnew2021b/Res ==
  res_msg : Inport
  function : TriggerPort  TriggerType=function-call  VariantControl=(inherit)
  Bus Selector : BusSelector  OutputSignals=res_stop
  Res_Msg : Subsystem
  res_signal : Outport
  res_error : Outport  Port=2
  wires:
  res_msg/1 -> Res_Msg/1(res_msg)
  Res_Msg/1(res_signal) -> Bus Selector/1, res_signal/1
  Bus Selector/1 -> res_error/1  "<res_stop>"

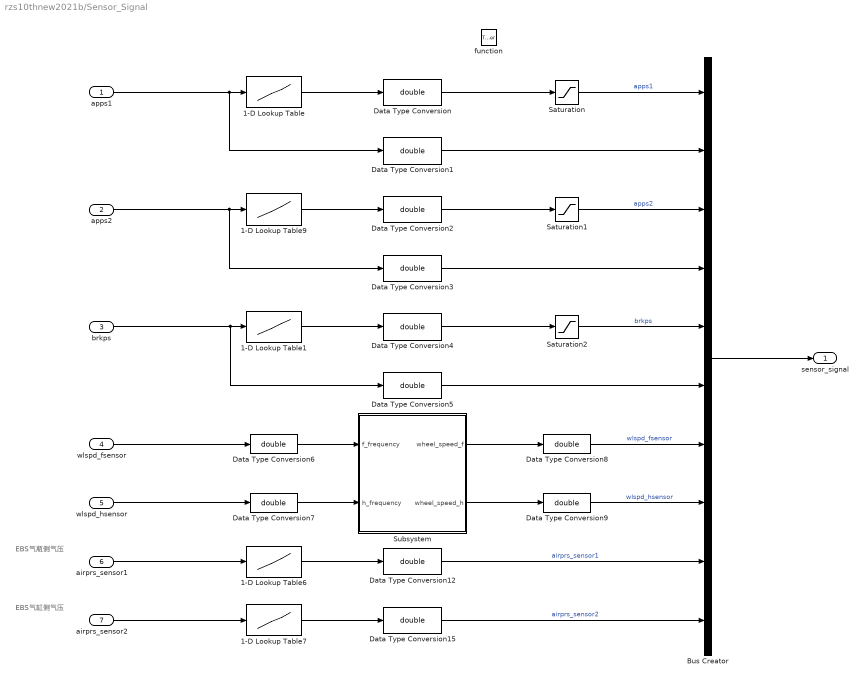
== system rzs10thnew2021b/Sensor_Signal ==
  note: EBS气缸侧气压
  note: EBS气瓶侧气压
  apps1 : Inport
  apps2 : Inport  Port=2
  brkps : Inport  Port=3
  wlspd_fsensor : Inport  Port=4
  wlspd_hsensor : Inport  Port=5
  airprs_sensor1 : Inport  Port=6
  airprs_sensor2 : Inport  Port=7
  function : TriggerPort  TriggerType=function-call  VariantControl=(inherit)
  1-D Lookup Table{,1,6..7,9} (5 alike) : Lookup_n-D  NumberOfTableDimensions=1  BreakpointsForDimension1=[252 2000]  IndexSearchMethod=Linear search  Table=[0 1]  ExtrapMethod=Clip  UseLastTableValue=on  InternalRulePriority=Speed  RndMeth=Simplest  InputSameDT=on
  Bus Creator : BusCreator  Inputs=10
  Data Type Conversion{,1..9,12,15} (12 alike) : DataTypeConversion  OutDataTypeStr=double
  Saturation : Saturate  UpperLimit=1  LowerLimit=0
  Saturation1 : Saturate  UpperLimit=1  LowerLimit=0
  Saturation2 : Saturate  UpperLimit=1  LowerLimit=0
  Subsystem : Subsystem
  sensor_signal : Outport
  wires:
  apps1/1 -> Data Type Conversion1/1, 1-D Lookup Table/1
  1-D Lookup Table/1 -> Data Type Conversion/1
  Data Type Conversion/1 -> Saturation/1
  Saturation/1 -> Bus Creator/1  "apps1"
  Data Type Conversion1/1 -> Bus Creator/2
  Data Type Conversion2/1 -> Saturation1/1
  apps2/1 -> 1-D Lookup Table9/1, Data Type Conversion3/1
  1-D Lookup Table9/1 -> Data Type Conversion2/1
  Saturation1/1 -> Bus Creator/3  "apps2"
  Data Type Conversion3/1 -> Bus Creator/4
  brkps/1 -> 1-D Lookup Table1/1, Data Type Conversion5/1
  1-D Lookup Table1/1 -> Data Type Conversion4/1
  Data Type Conversion4/1 -> Saturation2/1
  Saturation2/1 -> Bus Creator/5  "brkps"
  Data Type Conversion5/1 -> Bus Creator/6
  wlspd_fsensor/1 -> Data Type Conversion6/1
  Data Type Conversion6/1 -> Subsystem/1(f_frequency)
  wlspd_hsensor/1 -> Data Type Conversion7/1
  Data Type Conversion7/1 -> Subsystem/2(h_frequency)
  Subsystem/1(wheel_speed_f) -> Data Type Conversion8/1
  Subsystem/2(wheel_speed_h) -> Data Type Conversion9/1
  Data Type Conversion8/1 -> Bus Creator/7  "wlspd_fsensor"
  Data Type Conversion9/1 -> Bus Creator/8  "wlspd_hsensor"
  Bus Creator/1 -> sensor_signal/1
  Data Type Conversion12/1 -> Bus Creator/9  "airprs_sensor1"
  1-D Lookup Table7/1 -> Data Type Conversion15/1
  Data Type Conversion15/1 -> Bus Creator/10  "airprs_sensor2"
  1-D Lookup Table6/1 -> Data Type Conversion12/1
  airprs_sensor2/1 -> 1-D Lookup Table7/1
  airprs_sensor1/1 -> 1-D Lookup Table6/1

== system rzs10thnew2021b/TS_Activation ==
  di8_out : Inport
  run_button : Inport  Port=2
  tsms_button : Inport  Port=3
  brake_on : Inport  Port=4
  ami_inspection_signal : Inport  Port=5
  di8_in : Inport  Port=6
  function : TriggerPort  TriggerType=function-call  VariantControl=(inherit)
  Chart : Stateflow chart  TreatAsAtomicUnit=on
  Chart1 : Stateflow chart  TreatAsAtomicUnit=on
  Chart2 : Stateflow chart  TreatAsAtomicUnit=on
  Logical Operator : Logic  Operator=NOT  AllPortsSameDT=off  OutDataTypeStr=boolean
  Logical Operator1 : Logic  Operator=NOT  AllPortsSameDT=off  OutDataTypeStr=boolean
  Logical Operator2 : Logic  Operator=NOT  AllPortsSameDT=off  OutDataTypeStr=boolean
  Switch : Switch  Criteria=u2 > Threshold
  ts : Outport
  di8 : Outport  Port=2
  run : Outport  Port=3
  ts_warning : Outport  Port=4  OutDataTypeStr=boolean
  wires:
  di8_out/1 -> Logical Operator/1
  run_button/1 -> Logical Operator1/1
  Logical Operator1/1 -> Chart1/1(run_button)
  Chart2/1(ts) -> ts/1
  Chart/1(di8) -> di8/1, Chart2/1(di8)  "di8"
  Chart1/1(run) -> run/1, Chart2/2(run)  "run"
  tsms_button/1 -> Chart2/3(tsms_button)
  brake_on/1 -> Chart2/4(brake_on)
  ami_inspection_signal/1 -> Switch/2
  di8_in/1 -> Logical Operator2/1
  Logical Operator/1 -> Switch/1
  Logical Operator2/1 -> Switch/3
  Switch/1 -> Chart/1(di8_button)
  Chart2/2(ts_warning) -> ts_warning/1
